simulink model "mVeh_fun_tbm_block_test"  (R2020a)
settings: configuration reference "config_10ms" (kept outside this file)
undefined symbols (not defined in the file or in its folder): Calib_tbmVeh_drCmdMcP_incRate, Calib_tbmVeh_drCmdMcP_tgt, Calib_tbmVeh_set1_x4, Calib_tbmVeh_set2_x4, Parm_tbmVeh_sig_max_numInvalid, Parm_tbmVeh_sig_tolerate_numInvalid
libraries: speedgoatlib_IO691 x4, simulink x2, canmsglib x2, lib_signals_to_nByteLayout_withCrc x2, lib_cal_CAN_msgCount x2
settings Model: SimulationMode=external  PauseTimes=49.73  NumberOfSteps=20  Creator=jianjun.gao  LastModifiedBy=bowen.zheng
settings ConfigSetRef: SourceName=config_10ms  SourceLocation=Base Workspace

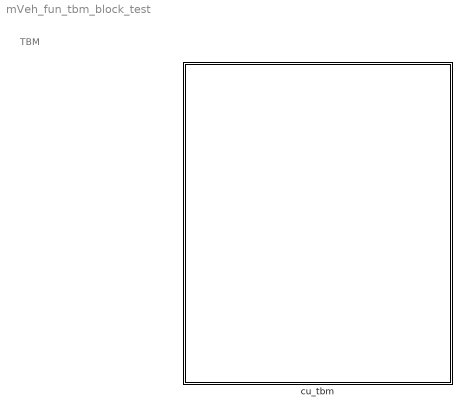
== system mVeh_fun_tbm_block_test ==
  note: TBM
  cu_tbm : Subsystem

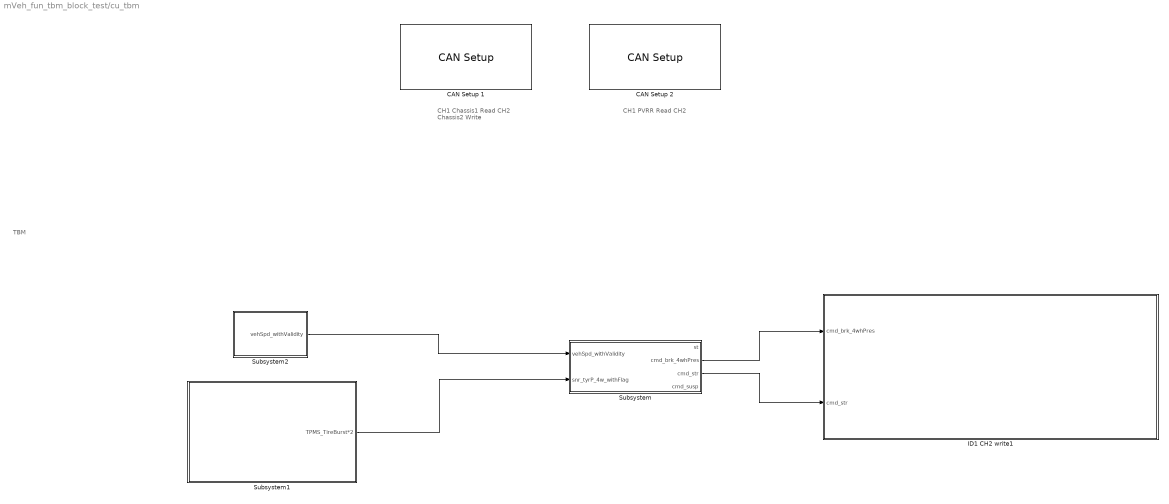
== system mVeh_fun_tbm_block_test/cu_tbm ==
  note: CH1 PVRR Read
      | CH2
  note: CH1 Chassis1 Read
      | CH2 Chassis2 Write
  note: TBM
  CAN Setup 1 : speedgoatlib_IO691/CAN Setup   moduletype=IO691  id=1  pciSlot=[12 0]  chn1=CAN (HS)  chn2=CAN (HS)  chn3=Disabled  chn4=Disabled  initStruct=[]  termStruct=[]  ArbitrationbdrChn1=500 kBaud  ArbitrationManbdrChn1=[2,16,63,16]  FdbdrChn1=5.0 MBaud  FdManbdrChn1=[2,2,5,2]  ArbitrationbdrChn2=500 kBaud  ArbitrationManbdrChn2=[2,16,63,16]  FdbdrChn2=5.0 MBaud  FdManbdrChn2=[2,2,5,2]  ArbitrationbdrChn3=1.0 MBaud  ArbitrationManbdrChn3=[2,8,31,8]  FdbdrChn3=5.0 MBaud  FdManbdrChn3=[2,2,5,2]  ArbitrationbdrChn4=1.0 MBaud  ArbitrationManbdrChn4=[2,8,31,8]  FdbdrChn4=5.0 MBaud  FdManbdrChn4=[2,2,5,2]  moduleInitValues=[691 1 12 0]
      settings: SourceProductName=Simulink Real-Time: Speedgoat I/O Blockset
  CAN Setup 2 : speedgoatlib_IO691/CAN Setup   moduletype=IO691  id=2  pciSlot=[7 0]  chn1=CAN (HS)  chn2=CAN (HS)  chn3=Disabled  chn4=Disabled  initStruct=[]  termStruct=[]  ArbitrationbdrChn1=500 kBaud  ArbitrationManbdrChn1=[2,16,63,16]  FdbdrChn1=5.0 MBaud  FdManbdrChn1=[2,2,5,2]  ArbitrationbdrChn2=500 kBaud  ArbitrationManbdrChn2=[2,16,63,16]  FdbdrChn2=5.0 MBaud  FdManbdrChn2=[2,2,5,2]  ArbitrationbdrChn3=1.0 MBaud  ArbitrationManbdrChn3=[2,8,31,8]  FdbdrChn3=5.0 MBaud  FdManbdrChn3=[2,2,5,2]  ArbitrationbdrChn4=1.0 MBaud  ArbitrationManbdrChn4=[2,8,31,8]  FdbdrChn4=5.0 MBaud  FdManbdrChn4=[2,2,5,2]  moduleInitValues=[691 2 7 0]
      settings: SourceProductName=Simulink Real-Time: Speedgoat I/O Blockset
  ID1 CH2 write1 : Subsystem
  Subsystem : Subsystem
  Subsystem1 : Subsystem
  Subsystem2 : Subsystem
  wires:
  ? -> ?
  Subsystem/3(cmd_str) -> ID1 CH2 write1/2(cmd_str)
  Subsystem/2(cmd_brk_4whPres) -> ID1 CH2 write1/1(cmd_brk_4whPres)
  Subsystem1/1(TPMS_TireBurst*2) -> Subsystem/2(snr_tyrP_4w_withFlag)
  Subsystem2/1(vehSpd_withValidity) -> Subsystem/1(vehSpd_withValidity)

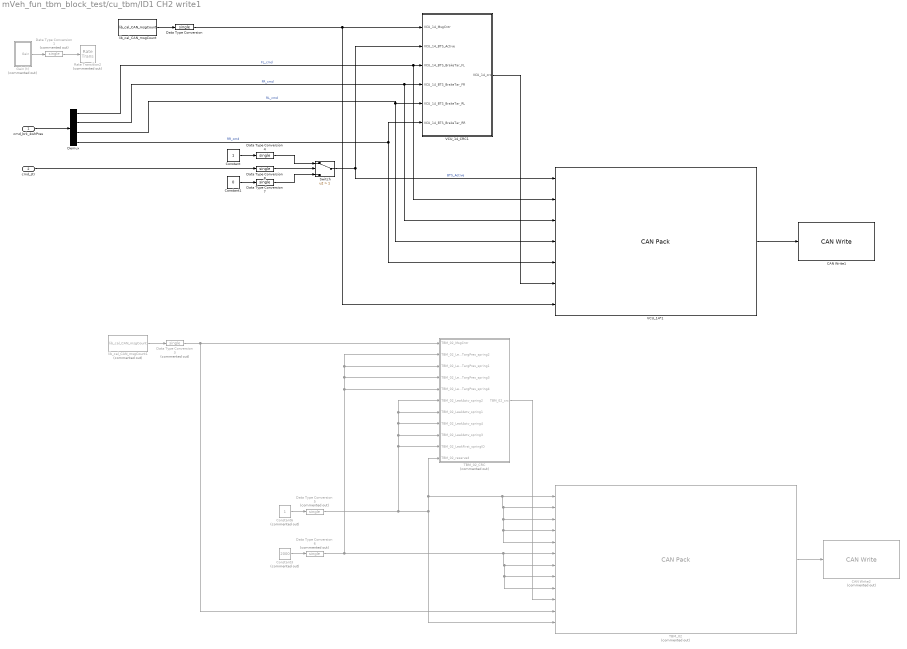
== system mVeh_fun_tbm_block_test/cu_tbm/ID1 CH2 write1 ==
  cmd_brk_4whPres : Inport
  cmd_str : Inport  Port=2
  CAN Write1 : speedgoatlib_IO691/CAN Write  id=1  ts=0.01  channel=2  messageType=CAN  enableStatusPort=off  canType=CAN (HS)  initValues=[691 1 0.01 1 1 1 0]
      settings: SourceProductName=Simulink Real-Time: Speedgoat I/O Blockset
  CAN Write2 : speedgoatlib_IO691/CAN Write  Commented=on  id=1  ts=0.01  channel=2  messageType=CAN  enableStatusPort=off  canType=CAN (HS)  initValues=[691 1 0.01 1 1 1 0]
      settings: SourceProductName=Simulink Real-Time: Speedgoat I/O Blockset
  Constant : Constant
  Constant1 : Constant  Value=0
  Constant3 : Constant  Commented=on  Value=2000
  Constant6 : Constant  Commented=on
  Data Type Conversion{,4,7..8} (4 alike) : DataTypeConversion  OutDataTypeStr=single
  Data Type Conversion{1,3,5..6} (4 alike) : DataTypeConversion  Commented=on  OutDataTypeStr=single
  Demux : Demux  Outputs=[1,1,1,1]
  Gain (t) : Subsystem  Commented=on
  Rate Transition2 : RateTransition  Commented=on
  Switch : Switch  Criteria=u2 > Threshold  Threshold=1
  TBM_02 : canmsglib/CAN Pack  Commented=on  CANdbFile=D:\spdGoat_prj_20221209\mVeh_fun_tbm_20221209\support\dbc\FCC1_NT2_Chassis1_CAN_Official_Release_V_1_4_DA_01_updated_mod.dbc  MsgList=(none)  MsgName=TBM_02  MsgIDType=Standard (11-bit identifier)  MsgIdentifier=128  MsgLength=8  Remote=off  ApplyMinMax=off  BusOutput=off  SignalInfo={'LeakActv_spring1','56','1','BE','unsigned','Standard','0','1','0','0','1';'LeakActv_spring2','57','1','BE','unsigned','Standard','0','1','0','0','1';'LeakActv_spring3','58','1','BE','unsigned','Standard','0','1','0','0','1';'LeakActv_spring4','59','1','BE','unsigned','Standard','0','1','0','0','1';'LeakFirst_springID','60','3','BE','unsigned','Standard','0','1','0','0','7';'LeakTargPres_spring1','17','11','BE','unsigned','Standard','0','1','0','0','2047';'LeakTargPres_spring2','38','11','BE','unsigned','Standard','0','1','0','0','2047';'LeakTargPres_spring3','43','11','BE','unsigned','Standard','0','1','0','0','2047';'LeakTargPres_spring4','48','11','BE','unsigned','Standard','0','1','0','0','2047';'TBM_02_CRC','0','8','BE','unsigned','Standard','0','1','0','0','255';'TBM_02_MsgCntr','12','4','BE','unsigned','Standard','0','1','0','0','15';'TBM_02_reserved','63','1','BE','unsigned','Standard','0','1','0','0','1'}
      settings: SourceProductBaseCode=ME,VN  DataFormat=CANdb specified signals
  TBM_02_CRC : Subsystem  Commented=on
  VCU_14*1 : canmsglib/CAN Pack  CANdbFile=D:\spdGoat_prj_20221209\mVeh_fun_tbm_20221209\support\dbc\NIO_NT2_Chassis2_CAN_Official_Release_V_1_1_DA_02.dbc  MsgList=(none)  MsgName=VCU_14  MsgIDType=Standard (11-bit identifier)  MsgIdentifier=75  MsgLength=8  Remote=off  ApplyMinMax=off  BusOutput=off  SignalInfo={'BTS_Active','23','1','BE','unsigned','Standard','0','1','0','0','1';'BTS_BrakeTar_FL','16','7','BE','unsigned','Standard','0','1','0','0','127';'BTS_BrakeTar_FR','25','7','BE','unsigned','Standard','0','1','0','0','127';'BTS_BrakeTar_RL','34','7','BE','unsigned','Standard','0','1','0','0','127';'BTS_BrakeTar_RR','43','7','BE','unsigned','Standard','0','1','0','0','127';'VCU_14_CRC','0','8','BE','unsigned','Standard','0','1','0','0','255';'VCU_14_MsgCntr','12','4','BE','unsigned','Standard','0','1','0','0','15'}
      settings: SourceProductBaseCode=ME,VN  DataFormat=CANdb specified signals
  VCU_14_CRC1 : Subsystem
  lib_cal_CAN_msgCount : lib_cal_CAN_msgCount/lib_cal_CAN_msgCount  SystemSampleTime=-1  Latency=0  AutoFrameSizeCalculation=off
  lib_cal_CAN_msgCount1 : lib_cal_CAN_msgCount/lib_cal_CAN_msgCount  Commented=on  SystemSampleTime=-1  Latency=0  AutoFrameSizeCalculation=off
  wires:
  Gain (t)/1("Gain ") -> Data Type Conversion1/1
  Constant/1 -> Data Type Conversion4/1
  Constant1/1 -> Data Type Conversion7/1
  Switch/1 -> VCU_14*1/1, VCU_14_CRC1/2("VCU_14_BTS_Active ")  "BTS_Active"
  VCU_14_CRC1/1(VCU_14_crc) -> VCU_14*1/6
  Data Type Conversion/1 -> VCU_14*1/7, VCU_14_CRC1/1("VCU_14_MsgCntr ")
  lib_cal_CAN_msgCount/1 -> Data Type Conversion/1
  VCU_14*1/1 -> CAN Write1/1
  Data Type Conversion1/1 -> Rate Transition2/1
  TBM_02/1 -> CAN Write2/1
  Constant6/1 -> Data Type Conversion5/1
  TBM_02_CRC/1(TBM_02_crc) -> TBM_02/10
  lib_cal_CAN_msgCount1/1 -> Data Type Conversion3/1
  Constant3/1 -> Data Type Conversion6/1
  Data Type Conversion6/1 -> TBM_02_CRC/5("TBM_02_LeakTargPres_spring4 "), TBM_02_CRC/4("TBM_02_LeakTargPres_spring3 "), TBM_02_CRC/3("TBM_02_LeakTargPres_spring1 "), TBM_02_CRC/2("TBM_02_LeakTargPres_spring2 "), TBM_02/9, TBM_02/8, TBM_02/7, TBM_02/6
  Data Type Conversion3/1 -> TBM_02/11, TBM_02_CRC/1("TBM_02_MsgCntr ")
  Data Type Conversion5/1 -> TBM_02_CRC/10(TBM_02_LeakFirst_springID), TBM_02_CRC/9(TBM_02_LeakActv_spring3), TBM_02_CRC/8("TBM_02_LeakActv_spring4 "), TBM_02_CRC/6(TBM_02_LeakActv_spring2), TBM_02_CRC/7("TBM_02_LeakActv_spring1 "), TBM_02/12, TBM_02_CRC/11(TBM_02_reserved), TBM_02/5, TBM_02/4, TBM_02/3, TBM_02/2, TBM_02/1
  Data Type Conversion4/1 -> Switch/1
  Data Type Conversion7/1 -> Switch/3
  cmd_str/1 -> Data Type Conversion8/1
  Data Type Conversion8/1 -> Switch/2
  Demux/1 -> VCU_14*1/2, VCU_14_CRC1/3("VCU_14_BTS_BrakeTar_FL ")  "FL_cmd"
  Demux/2 -> VCU_14_CRC1/4("VCU_14_BTS_BrakeTar_FR "), VCU_14*1/3  "FR_cmd"
  Demux/3 -> VCU_14*1/4, VCU_14_CRC1/5("VCU_14_BTS_BrakeTar_RL ")  "RL_cmd"
  Demux/4 -> VCU_14_CRC1/6("VCU_14_BTS_BrakeTar_RR "), VCU_14*1/5  "RR_cmd"
  cmd_brk_4whPres/1 -> Demux/1

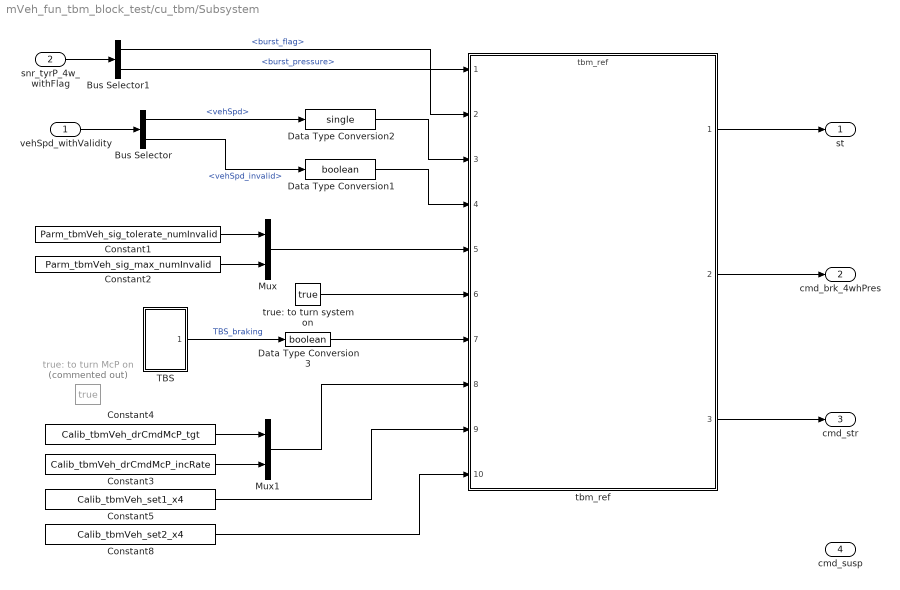
== system mVeh_fun_tbm_block_test/cu_tbm/Subsystem ==
  vehSpd_withValidity : Inport
  snr_tyrP_4w_withFlag : Inport  Port=2
  Bus Selector : BusSelector  OutputSignals=vehSpd,vehSpd_invalid
  Bus Selector1 : BusSelector  OutputSignals=burst_flag,burst_pressure
  Constant1 : Constant  Value=Parm_tbmVeh_sig_tolerate_numInvalid  OutDataTypeStr=int8  SampleTime=-1
  Constant2 : Constant  Value=Parm_tbmVeh_sig_max_numInvalid  OutDataTypeStr=int8  SampleTime=-1
  Constant3 : Constant  Value=Calib_tbmVeh_drCmdMcP_incRate  OutDataTypeStr=single  SampleTime=-1
  Constant4 : Constant  Value=Calib_tbmVeh_drCmdMcP_tgt  OutDataTypeStr=single  SampleTime=-1
  Constant5 : Constant  Value=Calib_tbmVeh_set1_x4  OutDataTypeStr=single  SampleTime=-1
  Constant8 : Constant  Value=Calib_tbmVeh_set2_x4  OutDataTypeStr=single  SampleTime=-1
  Data Type Conversion1 : DataTypeConversion  OutDataTypeStr=boolean
  Data Type Conversion2 : DataTypeConversion  OutDataTypeStr=single
  Data Type Conversion3 : DataTypeConversion  OutDataTypeStr=boolean
  Mux : Mux  Inputs=2
  Mux1 : Mux  Inputs=2
  TBS : Subsystem
  tbm_ref : ModelReference  ModelNameDialog=tbm_ref.slx  SimulationMode=Normal  ModelReferenceVersion=1.722
  true: to turn McP on : Constant  Commented=on  Value=true  OutDataTypeStr=boolean  SampleTime=-1
  true: to turn system on : Constant  Value=true  OutDataTypeStr=boolean  SampleTime=-1
  st : Outport
  cmd_brk_4whPres : Outport  Port=2
  cmd_str : Outport  Port=3
  cmd_susp : Outport  Port=4
  wires:
  Constant8/1 -> tbm_ref/10
  Data Type Conversion1/1 -> tbm_ref/4
  Mux1/1 -> tbm_ref/8
  Data Type Conversion2/1 -> tbm_ref/3
  Constant1/1 -> Mux/1
  Mux/1 -> tbm_ref/5
  Constant2/1 -> Mux/2
  tbm_ref/3 -> cmd_str/1
  Constant3/1 -> Mux1/2
  Constant4/1 -> Mux1/1
  tbm_ref/1 -> st/1
  Constant5/1 -> tbm_ref/9
  tbm_ref/2 -> cmd_brk_4whPres/1
  TBS/1("TBS_control ") -> Data Type Conversion3/1  "TBS_braking"
  Data Type Conversion3/1 -> tbm_ref/7
  snr_tyrP_4w_withFlag/1 -> Bus Selector1/1
  vehSpd_withValidity/1 -> Bus Selector/1
  Bus Selector/1 -> Data Type Conversion2/1  "<vehSpd>"
  Bus Selector/2 -> Data Type Conversion1/1  "<vehSpd_invalid>"
  Bus Selector1/2 -> tbm_ref/1  "<burst_pressure>"
  Bus Selector1/1 -> tbm_ref/2  "<burst_flag>"
  true: to turn system on/1 -> tbm_ref/6

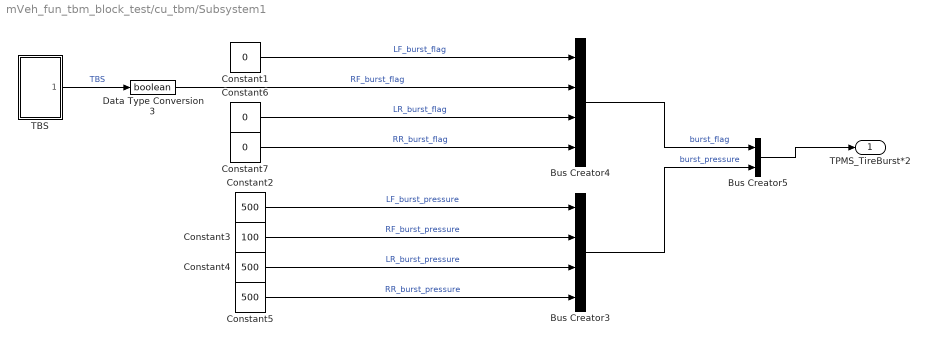
== system mVeh_fun_tbm_block_test/cu_tbm/Subsystem1 ==
  Bus Creator3 : BusCreator  Inputs=4
  Bus Creator4 : BusCreator  Inputs=4
  Bus Creator5 : BusCreator  Inputs=2
  Constant1 : Constant  Value=0  OutDataTypeStr=boolean
  Constant2 : Constant  Value=500  OutDataTypeStr=single
  Constant3 : Constant  Value=100  OutDataTypeStr=single
  Constant4 : Constant  Value=500  OutDataTypeStr=single
  Constant5 : Constant  Value=500  OutDataTypeStr=single
  Constant6 : Constant  Value=0  OutDataTypeStr=boolean
  Constant7 : Constant  Value=0  OutDataTypeStr=boolean
  Data Type Conversion3 : DataTypeConversion  OutDataTypeStr=boolean
  TBS : Subsystem
  TPMS_TireBurst*2 : Outport
  wires:
  Constant3/1 -> Bus Creator3/2  "RF_burst_pressure"
  Bus Creator5/1 -> TPMS_TireBurst*2/1
  Constant2/1 -> Bus Creator3/1  "LF_burst_pressure"
  Bus Creator4/1 -> Bus Creator5/1  "burst_flag"
  Bus Creator3/1 -> Bus Creator5/2  "burst_pressure"
  Constant1/1 -> Bus Creator4/1  "LF_burst_flag"
  Data Type Conversion3/1 -> Bus Creator4/2  "RF_burst_flag"
  TBS/1("TBS_control ") -> Data Type Conversion3/1  "TBS"
  Constant4/1 -> Bus Creator3/3  "LR_burst_pressure"
  Constant5/1 -> Bus Creator3/4  "RR_burst_pressure"
  Constant6/1 -> Bus Creator4/3  "LR_burst_flag"
  Constant7/1 -> Bus Creator4/4  "RR_burst_flag"

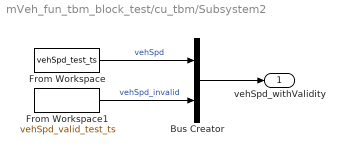
== system mVeh_fun_tbm_block_test/cu_tbm/Subsystem2 ==
  Bus Creator : BusCreator  Inputs=2
  From Workspace : FromWorkspace  VariableName=vehSpd_test_ts
  From Workspace1 : FromWorkspace  VariableName=vehSpd_valid_test_ts
  vehSpd_withValidity : Outport
  wires:
  Bus Creator/1 -> vehSpd_withValidity/1
  From Workspace/1 -> Bus Creator/1  "vehSpd"
  From Workspace1/1 -> Bus Creator/2  "vehSpd_invalid"

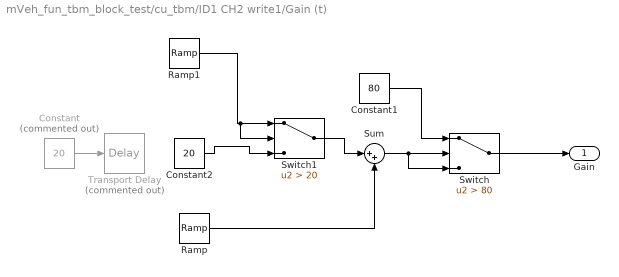
== system mVeh_fun_tbm_block_test/cu_tbm/ID1 CH2 write1/Gain (t) ==
  Constant : Constant  Commented=on  Value=20
  Constant1 : Constant  Value=80
  Constant2 : Constant  Value=20
  Ramp : simulink/Sources/Ramp  slope=60  start=20  InitialOutput=0
  Ramp1 : simulink/Sources/Ramp  slope=-600  start=10  InitialOutput=80
  Sum : Sum  Inputs=|++
  Switch : Switch  Criteria=u2 > Threshold  Threshold=80
  Switch1 : Switch  Criteria=u2 > Threshold  Threshold=20
  Transport Delay : TransportDelay  Commented=on  DelayTime=10  InitialOutput=80
  "Gain " : Outport
  wires:
  Constant1/1 -> Switch/1
  Ramp/1 -> Sum/2
  Sum/1 -> Switch/3, Switch/2
  Switch/1 -> "Gain "/1
  Constant/1 -> Transport Delay/1
  Ramp1/1 -> Switch1/2, Switch1/1
  Constant2/1 -> Switch1/3
  Switch1/1 -> Sum/1

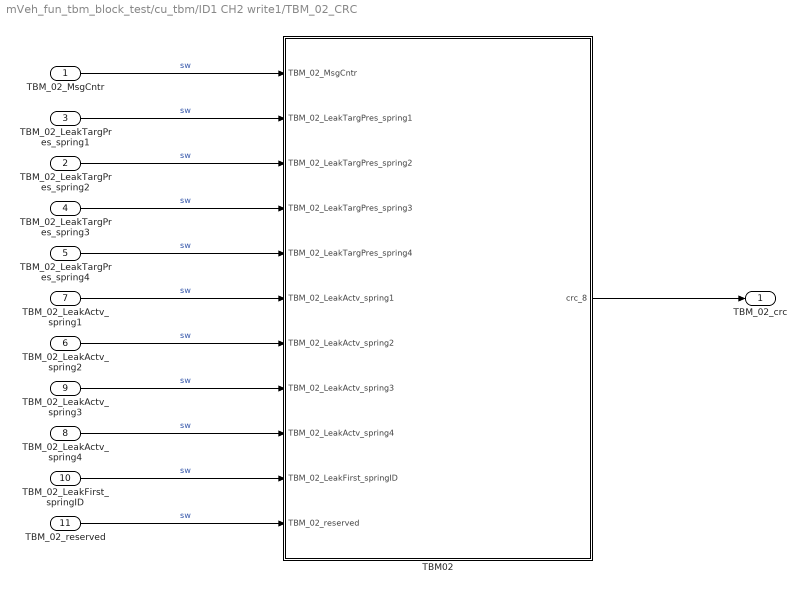
== system mVeh_fun_tbm_block_test/cu_tbm/ID1 CH2 write1/TBM_02_CRC ==
  "TBM_02_MsgCntr " : Inport
  "TBM_02_LeakTargPres_spring2 " : Inport  Port=2
  "TBM_02_LeakTargPres_spring1 " : Inport  Port=3
  "TBM_02_LeakTargPres_spring3 " : Inport  Port=4
  "TBM_02_LeakTargPres_spring4 " : Inport  Port=5
  TBM_02_LeakActv_spring2 : Inport  Port=6
  "TBM_02_LeakActv_spring1 " : Inport  Port=7
  "TBM_02_LeakActv_spring4 " : Inport  Port=8
  TBM_02_LeakActv_spring3 : Inport  Port=9
  TBM_02_LeakFirst_springID : Inport  Port=10
  TBM_02_reserved : Inport  Port=11
  TBM02 : Subsystem
  TBM_02_crc : Outport
  wires:
  "TBM_02_LeakTargPres_spring4 "/1 -> TBM02/5("TBM_02_LeakTargPres_spring4 ")  "sw"
  "TBM_02_LeakActv_spring1 "/1 -> TBM02/6("TBM_02_LeakActv_spring1 ")  "sw"
  "TBM_02_MsgCntr "/1 -> TBM02/1("TBM_02_MsgCntr ")  "sw"
  "TBM_02_LeakTargPres_spring1 "/1 -> TBM02/2("TBM_02_LeakTargPres_spring1 ")  "sw"
  "TBM_02_LeakTargPres_spring2 "/1 -> TBM02/3("TBM_02_LeakTargPres_spring2 ")  "sw"
  "TBM_02_LeakTargPres_spring3 "/1 -> TBM02/4("TBM_02_LeakTargPres_spring3 ")  "sw"
  TBM02/1(crc_8) -> TBM_02_crc/1
  "TBM_02_LeakActv_spring4 "/1 -> TBM02/9("TBM_02_LeakActv_spring4 ")  "sw"
  TBM_02_LeakActv_spring3/1 -> TBM02/8("TBM_02_LeakActv_spring3 ")  "sw"
  TBM_02_LeakActv_spring2/1 -> TBM02/7(TBM_02_LeakActv_spring2)  "sw"
  TBM_02_reserved/1 -> TBM02/11("TBM_02_reserved ")  "sw"
  TBM_02_LeakFirst_springID/1 -> TBM02/10(TBM_02_LeakFirst_springID)  "sw"

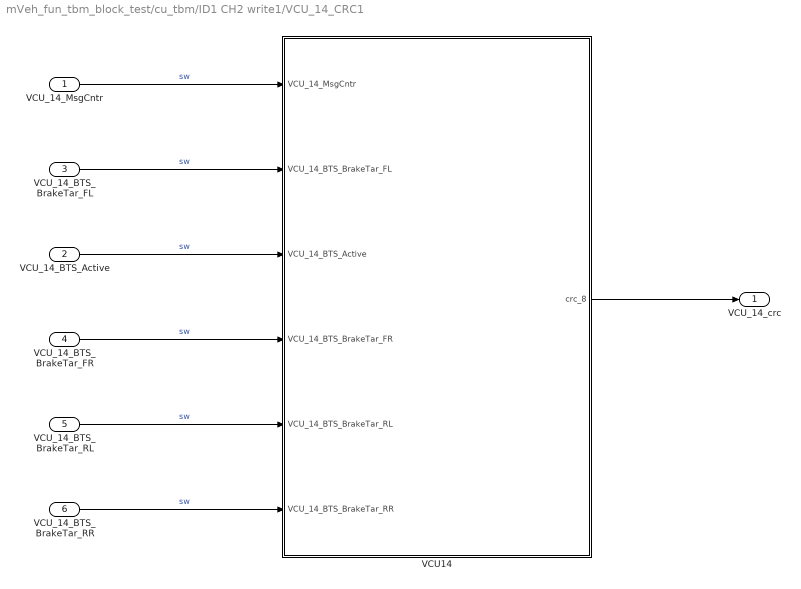
== system mVeh_fun_tbm_block_test/cu_tbm/ID1 CH2 write1/VCU_14_CRC1 ==
  "VCU_14_MsgCntr " : Inport
  "VCU_14_BTS_Active " : Inport  Port=2
  "VCU_14_BTS_BrakeTar_FL " : Inport  Port=3
  "VCU_14_BTS_BrakeTar_FR " : Inport  Port=4
  "VCU_14_BTS_BrakeTar_RL " : Inport  Port=5
  "VCU_14_BTS_BrakeTar_RR " : Inport  Port=6
  VCU14 : Subsystem
  VCU_14_crc : Outport
  wires:
  "VCU_14_BTS_BrakeTar_RL "/1 -> VCU14/5("VCU_14_BTS_BrakeTar_RL ")  "sw"
  "VCU_14_BTS_BrakeTar_RR "/1 -> VCU14/6("VCU_14_BTS_BrakeTar_RR ")  "sw"
  "VCU_14_MsgCntr "/1 -> VCU14/1("VCU_14_MsgCntr ")  "sw"
  "VCU_14_BTS_BrakeTar_FL "/1 -> VCU14/2("VCU_14_BTS_BrakeTar_FL ")  "sw"
  "VCU_14_BTS_Active "/1 -> VCU14/3("VCU_14_BTS_Active ")  "sw"
  "VCU_14_BTS_BrakeTar_FR "/1 -> VCU14/4("VCU_14_BTS_BrakeTar_FR ")  "sw"
  VCU14/1(crc_8) -> VCU_14_crc/1

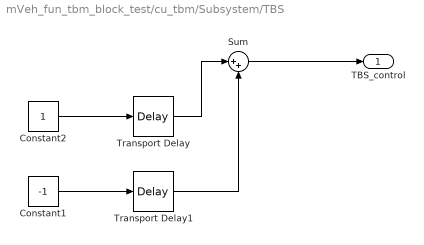
== system mVeh_fun_tbm_block_test/cu_tbm/Subsystem/TBS ==
  Constant1 : Constant  Value=-1
  Constant2 : Constant
  Sum : Sum  Inputs=|++
  Transport Delay : TransportDelay  DelayTime=3
  Transport Delay1 : TransportDelay  DelayTime=10
  "TBS_control " : Outport
  wires:
  Constant2/1 -> Transport Delay/1
  Transport Delay/1 -> Sum/1
  Sum/1 -> "TBS_control "/1
  Constant1/1 -> Transport Delay1/1
  Transport Delay1/1 -> Sum/2

== system mVeh_fun_tbm_block_test/cu_tbm/Subsystem1/TBS ==
  Constant2 : Constant
  Transport Delay : TransportDelay
  "TBS_control " : Outport
  wires:
  Constant2/1 -> Transport Delay/1
  Transport Delay/1 -> "TBS_control "/1

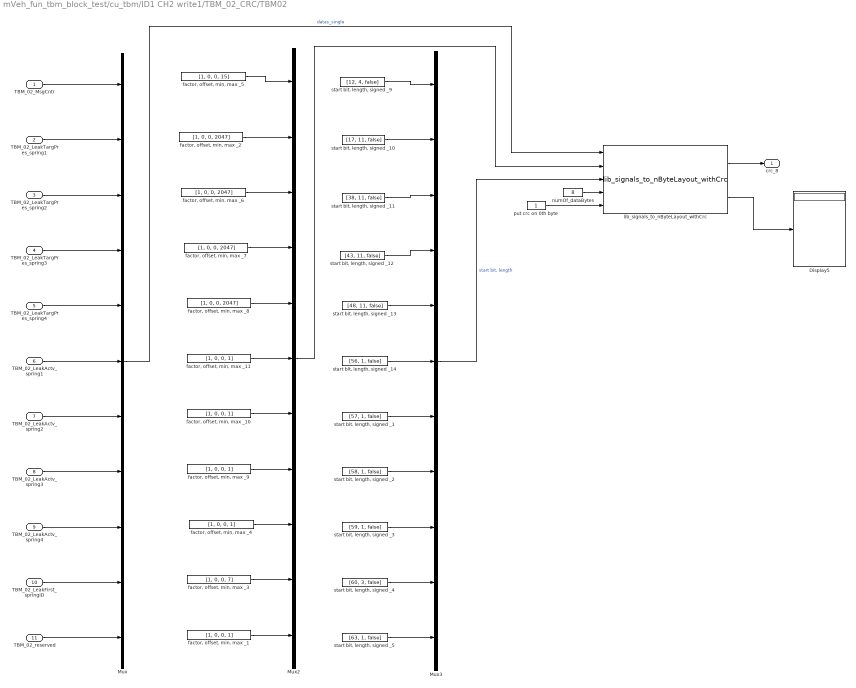
== system mVeh_fun_tbm_block_test/cu_tbm/ID1 CH2 write1/TBM_02_CRC/TBM02 ==
  "TBM_02_MsgCntr " : Inport
  "TBM_02_LeakTargPres_spring1 " : Inport  Port=2
  "TBM_02_LeakTargPres_spring2 " : Inport  Port=3
  "TBM_02_LeakTargPres_spring3 " : Inport  Port=4
  "TBM_02_LeakTargPres_spring4 " : Inport  Port=5
  "TBM_02_LeakActv_spring1 " : Inport  Port=6
  TBM_02_LeakActv_spring2 : Inport  Port=7
  "TBM_02_LeakActv_spring3 " : Inport  Port=8
  "TBM_02_LeakActv_spring4 " : Inport  Port=9
  TBM_02_LeakFirst_springID : Inport  Port=10
  "TBM_02_reserved " : Inport  Port=11
  Display5 : Display
  Mux : Mux  Inputs=11
  Mux2 : Mux  Inputs=11
  Mux3 : Mux  Inputs=11
  factor, offset, min, max _{1,4,9..11} (5 alike) : Constant  Value=[1, 0, 0, 1]  OutDataTypeStr=single  SampleTime=-1
  factor, offset, min, max _{2,6..8} (4 alike) : Constant  Value=[1, 0, 0, 2047]  OutDataTypeStr=single  SampleTime=-1
  "factor, offset, min, max _3" : Constant  Value=[1, 0, 0, 7]  OutDataTypeStr=single  SampleTime=-1
  "factor, offset, min, max _5" : Constant  Value=[1, 0, 0, 15]  OutDataTypeStr=single  SampleTime=-1
  lib_signals_to_nByteLayout_withCrc : lib_signals_to_nByteLayout_withCrc/lib_signals_to_nByteLayout_withCrc  SystemSampleTime=-1  Latency=0  AutoFrameSizeCalculation=off
  numOf_dataBytes : Constant  Value=8  OutDataTypeStr=uint8  SampleTime=-1
  put crc on 0th byte : Constant  OutDataTypeStr=uint8  SampleTime=-1
  "start bit, length, signed _1" : Constant  Value=[57, 1, false]  OutDataTypeStr=uint8  SampleTime=-1
  "start bit, length, signed _10" : Constant  Value=[17, 11, false]  OutDataTypeStr=uint8  SampleTime=-1
  "start bit, length, signed _11" : Constant  Value=[38, 11, false]  OutDataTypeStr=uint8  SampleTime=-1
  "start bit, length, signed _12" : Constant  Value=[43, 11, false]  OutDataTypeStr=uint8  SampleTime=-1
  "start bit, length, signed _13" : Constant  Value=[48, 11, false]  OutDataTypeStr=uint8  SampleTime=-1
  "start bit, length, signed _14" : Constant  Value=[56, 1, false]  OutDataTypeStr=uint8  SampleTime=-1
  "start bit, length, signed _2" : Constant  Value=[58, 1, false]  OutDataTypeStr=uint8  SampleTime=-1
  "start bit, length, signed _3" : Constant  Value=[59, 1, false]  OutDataTypeStr=uint8  SampleTime=-1
  "start bit, length, signed _4" : Constant  Value=[60, 3, false]  OutDataTypeStr=uint8  SampleTime=-1
  "start bit, length, signed _5" : Constant  Value=[63, 1, false]  OutDataTypeStr=uint8  SampleTime=-1
  "start bit, length, signed _9" : Constant  Value=[12, 4, false]  OutDataTypeStr=uint8  SampleTime=-1
  crc_8 : Outport
  wires:
  "TBM_02_LeakTargPres_spring1 "/1 -> Mux/2
  "TBM_02_LeakTargPres_spring4 "/1 -> Mux/5
  "start bit, length, signed _12"/1 -> Mux3/4
  Mux/1 -> lib_signals_to_nByteLayout_withCrc/1  "datas_single"
  "start bit, length, signed _13"/1 -> Mux3/5
  "TBM_02_MsgCntr "/1 -> Mux/1
  "TBM_02_LeakTargPres_spring3 "/1 -> Mux/4
  "start bit, length, signed _11"/1 -> Mux3/3
  "start bit, length, signed _9"/1 -> Mux3/1
  lib_signals_to_nByteLayout_withCrc/2 -> Display5/1
  "start bit, length, signed _14"/1 -> Mux3/6
  "TBM_02_LeakTargPres_spring2 "/1 -> Mux/3
  Mux3/1 -> lib_signals_to_nByteLayout_withCrc/3  "start bit, length"
  "factor, offset, min, max _2"/1 -> Mux2/2
  put crc on 0th byte/1 -> lib_signals_to_nByteLayout_withCrc/5
  "factor, offset, min, max _6"/1 -> Mux2/3
  "factor, offset, min, max _5"/1 -> Mux2/1
  Mux2/1 -> lib_signals_to_nByteLayout_withCrc/2
  "start bit, length, signed _10"/1 -> Mux3/2
  "TBM_02_LeakActv_spring1 "/1 -> Mux/6
  lib_signals_to_nByteLayout_withCrc/1 -> crc_8/1
  numOf_dataBytes/1 -> lib_signals_to_nByteLayout_withCrc/4
  "factor, offset, min, max _7"/1 -> Mux2/4
  "factor, offset, min, max _8"/1 -> Mux2/5
  "factor, offset, min, max _11"/1 -> Mux2/6
  TBM_02_LeakActv_spring2/1 -> Mux/7
  "TBM_02_LeakActv_spring3 "/1 -> Mux/8
  TBM_02_LeakFirst_springID/1 -> Mux/10
  "TBM_02_reserved "/1 -> Mux/11
  "TBM_02_LeakActv_spring4 "/1 -> Mux/9
  "factor, offset, min, max _1"/1 -> Mux2/11
  "factor, offset, min, max _3"/1 -> Mux2/10
  "factor, offset, min, max _4"/1 -> Mux2/9
  "factor, offset, min, max _9"/1 -> Mux2/8
  "factor, offset, min, max _10"/1 -> Mux2/7
  "start bit, length, signed _1"/1 -> Mux3/7
  "start bit, length, signed _2"/1 -> Mux3/8
  "start bit, length, signed _3"/1 -> Mux3/9
  "start bit, length, signed _4"/1 -> Mux3/10
  "start bit, length, signed _5"/1 -> Mux3/11

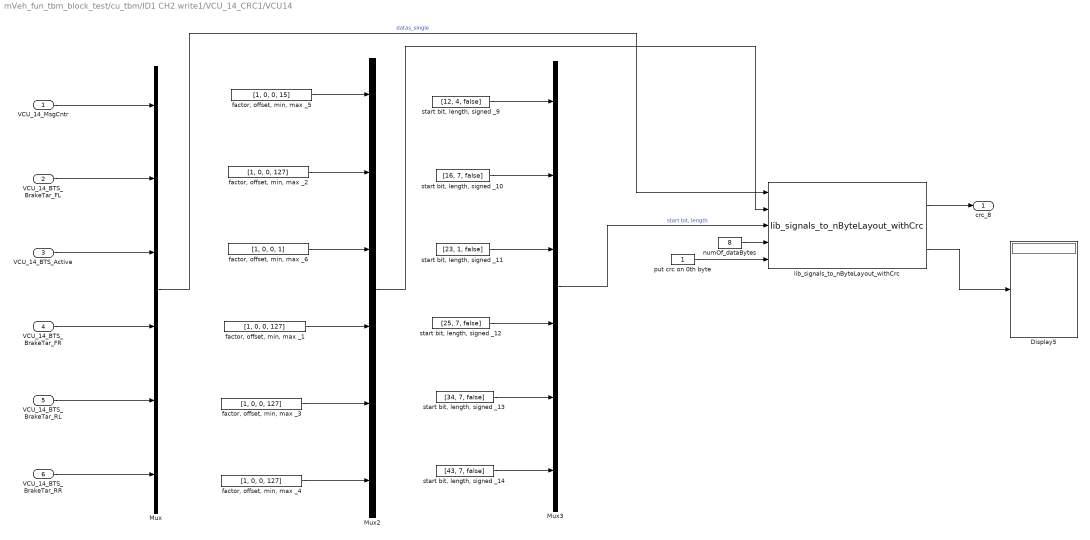
== system mVeh_fun_tbm_block_test/cu_tbm/ID1 CH2 write1/VCU_14_CRC1/VCU14 ==
  "VCU_14_MsgCntr " : Inport
  "VCU_14_BTS_BrakeTar_FL " : Inport  Port=2
  "VCU_14_BTS_Active " : Inport  Port=3
  "VCU_14_BTS_BrakeTar_FR " : Inport  Port=4
  "VCU_14_BTS_BrakeTar_RL " : Inport  Port=5
  "VCU_14_BTS_BrakeTar_RR " : Inport  Port=6
  Display5 : Display
  Mux : Mux  Inputs=6
  Mux2 : Mux  Inputs=6
  Mux3 : Mux  Inputs=6
  factor, offset, min, max _{1..4} (4 alike) : Constant  Value=[1, 0, 0, 127]  OutDataTypeStr=single  SampleTime=-1
  "factor, offset, min, max _5" : Constant  Value=[1, 0, 0, 15]  OutDataTypeStr=single  SampleTime=-1
  "factor, offset, min, max _6" : Constant  Value=[1, 0, 0, 1]  OutDataTypeStr=single  SampleTime=-1
  lib_signals_to_nByteLayout_withCrc : lib_signals_to_nByteLayout_withCrc/lib_signals_to_nByteLayout_withCrc  SystemSampleTime=-1  Latency=0  AutoFrameSizeCalculation=off
  numOf_dataBytes : Constant  Value=8  OutDataTypeStr=uint8  SampleTime=-1
  put crc on 0th byte : Constant  OutDataTypeStr=uint8  SampleTime=-1
  "start bit, length, signed _10" : Constant  Value=[16, 7, false]  OutDataTypeStr=uint8  SampleTime=-1
  "start bit, length, signed _11" : Constant  Value=[23, 1, false]  OutDataTypeStr=uint8  SampleTime=-1
  "start bit, length, signed _12" : Constant  Value=[25, 7, false]  OutDataTypeStr=uint8  SampleTime=-1
  "start bit, length, signed _13" : Constant  Value=[34, 7, false]  OutDataTypeStr=uint8  SampleTime=-1
  "start bit, length, signed _14" : Constant  Value=[43, 7, false]  OutDataTypeStr=uint8  SampleTime=-1
  "start bit, length, signed _9" : Constant  Value=[12, 4, false]  OutDataTypeStr=uint8  SampleTime=-1
  crc_8 : Outport
  wires:
  "VCU_14_BTS_BrakeTar_FL "/1 -> Mux/2
  "VCU_14_BTS_BrakeTar_RL "/1 -> Mux/5
  "start bit, length, signed _12"/1 -> Mux3/4
  Mux/1 -> lib_signals_to_nByteLayout_withCrc/1  "datas_single"
  "start bit, length, signed _13"/1 -> Mux3/5
  "VCU_14_MsgCntr "/1 -> Mux/1
  "VCU_14_BTS_BrakeTar_FR "/1 -> Mux/4
  "start bit, length, signed _11"/1 -> Mux3/3
  "start bit, length, signed _9"/1 -> Mux3/1
  lib_signals_to_nByteLayout_withCrc/2 -> Display5/1
  "start bit, length, signed _14"/1 -> Mux3/6
  "VCU_14_BTS_Active "/1 -> Mux/3
  Mux3/1 -> lib_signals_to_nByteLayout_withCrc/3  "start bit, length"
  "factor, offset, min, max _2"/1 -> Mux2/2
  put crc on 0th byte/1 -> lib_signals_to_nByteLayout_withCrc/5
  "factor, offset, min, max _6"/1 -> Mux2/3
  "factor, offset, min, max _5"/1 -> Mux2/1
  Mux2/1 -> lib_signals_to_nByteLayout_withCrc/2
  "start bit, length, signed _10"/1 -> Mux3/2
  "VCU_14_BTS_BrakeTar_RR "/1 -> Mux/6
  lib_signals_to_nByteLayout_withCrc/1 -> crc_8/1
  numOf_dataBytes/1 -> lib_signals_to_nByteLayout_withCrc/4
  "factor, offset, min, max _1"/1 -> Mux2/4
  "factor, offset, min, max _3"/1 -> Mux2/5
  "factor, offset, min, max _4"/1 -> Mux2/6
